simulink model "stellaris_extmode"  (R2014b)
settings: Solver=FixedStepDiscrete  StartTime=0.0  StopTime=10.0  RelTol=1e-3
PreLoadFcn:
  | RTWConfigurationCB('preloadfcn', bdroot);
libraries: stellaris_lib x3, driver_interface_library x2, canblocks_extras x1, targetsExternalModeSwitchLib x1
settings Model: SimulationMode=external  Creator=bas  LastModifiedBy=peselnikmg
settings OptimizationCC: InlineParams=on  OptimizeModelRefInitCode=on  LifeSpan=1
settings DebuggingCC: UnderspecifiedInitializationDetection=Classic  MergeDetectMultiDrivingBlocksExec=none  StateNameClashWarn=warning
settings HardwareCC: ProdEndianess=LittleEndian  ProdHWDeviceType=Texas Instruments->TMS470
settings RTWCC: SystemTargetFile=stellaris.tlc  TemplateMakefile=stellaris_tmf  PostCodeGenCommand=stellaris_customcode(buildInfo)  Description=TI Stellaris LaunchPad  GenerateReport=on  ProcessScript=stellaris_make_rtw_hook  IncludeHyperlinkInReport=on  GenerateTraceInfo=on  GenerateTraceReport=on  GenerateTraceReportSl=on  GenerateTraceReportSf=on  GenerateTraceReportEml=on
settings CodeAppCC: IgnoreCustomStorageClasses=off
settings STFCustomTargetCC: CombineOutputUpdateFcns=on  ERTCustomFileBanners=on  SupportContinuousTime=off  SupportNonInlinedSFcns=off  MATLABClassNameForMDSCustomization=Simulink.SoftwareTarget.ERTCustomization  GRTInterface=off  SystemTargetFile=stellaris.tlc
settings ERTTargetCC: ParMdlRefBuildCompliant=off  CompOptLevelCompliant=off  ConcurrentExecutionCompliant=off  ERTFirstTimeCompliant=off  ModelStepFunctionPrototypeControlCompliant=off  CPPClassGenCompliant=off  GenerateASAP2=on  ExtMode=on  ExtModeTransport=1  ExtModeStaticAllocSize=25000  ExtModeMexFile=stellarisExternalModeOpen  ExtModeMexArgs=1 getpref('stellaris','COMPort') 115200  ExtModeIntrfLevel=Level2  InlinedParameterPlacement=NonHierarchical  ERTCustomFileTemplate=stellaris_main.tlc

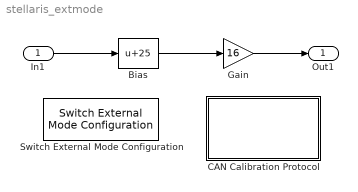
== system stellaris_extmode ==
  In1 : Inport
  Bias : Bias  Bias=25
  CAN Calibration Protocol : Subsystem  InitFcn=|  mask(Stellaris CAN Calibration Protocol){CCP_STATION_ID=hex2dec('1'), module=eCAN_A, ccp_cro_id=hex2dec('6FA'), ccp_cro_message_type=Extended (29-bit identifier), ccp_return_id=hex2dec('6FB'), ccp_return_message_type=Extended (29-bit identifier), TOTAL_NUM_ODTS=8, cro_sample_time=0.1}
      | % START RTW CONFIGURATION CODE %
      | RTWConfigurationCB('rtw_target_initfcn',gcb);
      | % END RTW CONFIGURATION CODE %
      mask prompts: CCP_STATION_ID "CCP station address (16-bit integer):"; module "CAN module:"; ccp_cro_id "CAN message identifier (CRO):"; ccp_cro_message_type "CAN message type (CRO):"; ccp_return_id "CAN message identifier (DTO/DAQ):"; ccp_return_message_type "CAN message type (DTO/DAQ):"; TOTAL_NUM_ODTS "Total Number of Object Descriptor Tables (ODTs):"; cro_sample_time "CRO sample time:"
      mask help:
      | Implements CAN Calibration Protocol (CCP) on the target processor.
      |
      | This block processes Command Receive Object (CRO) messages and outputs the resulting Data Transmission Object (DTO) and Data Acquisition (DAQ) messages.
      mask init:
      | % % Propagate DAQ / DTO message type to underlying blocks
      | % set_param([gcb, '/DAQ Processing/Send DAQ Message/eCAN Transmit'], 'messageType', ccp_return_message_type);
      | % set_param([gcb, '/DTO Processing/CCP(Termination)/CAN Transmit/eCAN Transmit'], 'messageType', ccp_return_message_type);
      | % % Propagate CRO message type to underlying blocks
      | % set_param([gcb, '/eCAN Receive'], 'messageType', ccp_cro_message_type);
      | % % Propagate eCAN module to underlying blocks
      | % set_param([gcb, '/DAQ Processing/Send DAQ Message/eCAN Transmit'], 'useModule', module);
      | % set_param([gcb, '/DTO Processing/CCP(Termination)/CAN Transmit/eCAN Transmit'], 'useModule', module);
      | % set_param([gcb, '/eCAN Receive'], 'useModule', module);
      mask Help: eval('codertarget.internal.helpView(''tic2000'' ,''c280xlibc28xcancalibrationprotocol'')')
      mask TypeOptions module: eCAN_A | eCAN_B
      mask TypeOptions ccp_cro_message_type: Standard (11-bit identifier) | Extended (29-bit identifier)
      mask TypeOptions ccp_return_message_type: Standard (11-bit identifier) | Extended (29-bit identifier)
      mask Display:
      | color('blue');
      | text(0.95, 0.90, 'C28x', ...
      |                 'horizontalalignment', 'right');
      | color('black');
      | text(0.50, 0.12, 'CCP', ...
      |                 'horizontalAlignment','center');
  Gain : Gain  Gain=16
  Switch External Mode Configuration : targetsExternalModeSwitchLib/Switch External Mode Configuration  SystemSampleTime=-1
  Out1 : Outport
  wires:
  In1/1 -> Bias/1
  Bias/1 -> Gain/1
  Gain/1 -> Out1/1

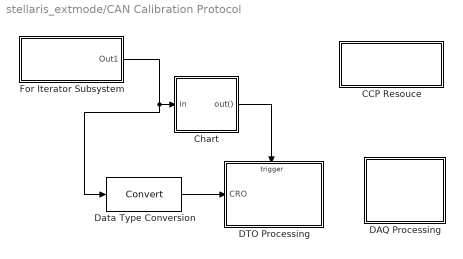
== system stellaris_extmode/CAN Calibration Protocol ==
  CCP Resouce : Subsystem  Tag=RTW CONFIGURATION BLOCK  Priority=-100000  mask{oldParentName=stellaris_extmode/CAN Calibration Protocol, oldBlockName=stellaris_extmode/CAN Calibration Protocol/CCP Resouce, defaultConfigLibrary=}
      mask prompts: oldParentName "Old Parent Name"; oldBlockName "Old Block Name"; defaultConfigLibrary "Default Config Library"
      settings: CopyFcn=RTWConfigurationCB('copyfcn',gcb);  DeleteFcn=RTWConfigurationCB('deletefcn',gcb);  UndoDeleteFcn=RTWConfigurationCB('NameChangeFcn',gcb);  PreSaveFcn=RTWConfigurationCB('presavefcn',gcb);  NameChangeFcn=RTWConfigurationCB('NameChangeFcn',gcb);  OpenFcn=RTWConfigurationCB('openfcn',gcb);
      mask Display: disp('CCP\nResource Block')
  Chart : Stateflow chart  TreatAsAtomicUnit=on
  DAQ Processing : Subsystem
      mask Display: disp('DAQ')
  DTO Processing : Subsystem
      mask Display: disp('DTO')
  Data Type Conversion : DataTypeConversion
  For Iterator Subsystem : Subsystem  TreatAsAtomicUnit=on
  wires:
  Data Type Conversion/1 -> DTO Processing/1(CRO)
  For Iterator Subsystem/1(Out1) -> Chart/1(in), Data Type Conversion/1
  Chart/1(out()) -> DTO Processing/Trigger

== system stellaris_extmode/CAN Calibration Protocol/CCP Resouce ==

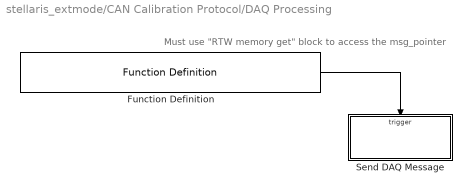
== system stellaris_extmode/CAN Calibration Protocol/DAQ Processing ==
  note: Must use "RTW memory get" block to access the msg_pointer
  Function Definition : driver_interface_library/Function Definition  function_name='void exported_ccp_daq_trigger(uint8_T * msg_pointer)'
  Send DAQ Message : Subsystem  TreatAsAtomicUnit=on
  wires:
  Function Definition/1 -> Send DAQ Message/Trigger

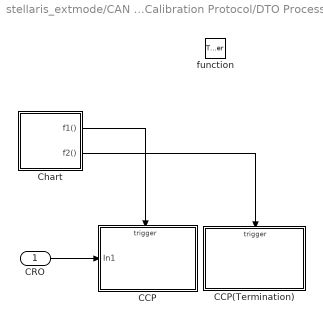
== system stellaris_extmode/CAN Calibration Protocol/DTO Processing ==
  CRO : Inport
  function : TriggerPort  TriggerType=function-call
  CCP : Subsystem
  CCP(Termination) : Subsystem
  Chart : Stateflow chart  TreatAsAtomicUnit=on
  wires:
  Chart/1(f1()) -> CCP/Trigger
  Chart/2(f2()) -> CCP(Termination)/Trigger
  CRO/1 -> CCP/1(In1)

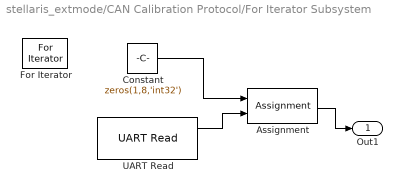
== system stellaris_extmode/CAN Calibration Protocol/For Iterator Subsystem ==
  Assignment : Assignment  OutputInitialize=Specify size for each dimension in table  DiagnosticForDimensions=Warning
  Constant : Constant  Value=zeros(1,8,'int32')
  For Iterator : ForIterator  IterationLimit=8  ShowIterationPort=off
  UART Read : stellaris_lib/UART/UART Read  nbFlag=on
  Out1 : Outport
  wires:
  UART Read/1 -> Assignment/2
  Assignment/1 -> Out1/1
  Constant/1 -> Assignment/1

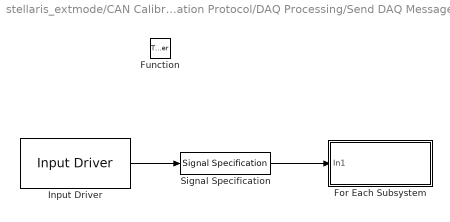
== system stellaris_extmode/CAN Calibration Protocol/DAQ Processing/Send DAQ Message ==
  Function : TriggerPort  TriggerType=function-call
  For Each Subsystem : Subsystem  TreatAsAtomicUnit=on
  Input Driver : driver_interface_library/Input Driver  t=-1  expr='msg_pointer[%<i>]'  portWidth=8  pOpt=[]  expression_type=Not expression
  Signal Specification : SignalSpecification  OutDataTypeStr=uint8
  wires:
  Input Driver/1 -> Signal Specification/1
  Signal Specification/1 -> For Each Subsystem/1(In1)

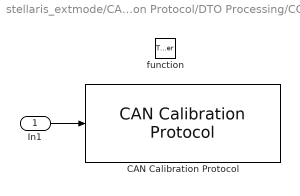
== system stellaris_extmode/CAN Calibration Protocol/DTO Processing/CCP ==
  In1 : Inport
  function : TriggerPort  TriggerType=function-call
  CAN Calibration Protocol : canblocks_extras/CAN Calibration Protocol  CCP_STATION_ID=CCP_STATION_ID  TOTAL_NUM_ODTS=TOTAL_NUM_ODTS  show_commands=off  GET_CCP_VERSIONenabled=on  EXCHANGE_IDenabled=on  SET_MTAenabled=on  DNLOADenabled=on  DNLOAD_6enabled=on  UPLOADenabled=on  SHORT_UPenabled=on  GET_DAQ_SIZEenabled=on  SET_DAQ_PTRenabled=on  WRITE_DAQenabled=on  START_STOPenabled=on  SET_S_STATUSenabled=on  GET_S_STATUSenabled=on  START_STOP_ALLenabled=on
      settings: AttributesFormatString=\n\n
  wires:
  In1/1 -> CAN Calibration Protocol/1

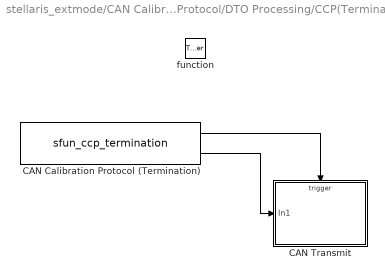
== system stellaris_extmode/CAN Calibration Protocol/DTO Processing/CCP(Termination) ==
  function : TriggerPort  TriggerType=function-call
  CAN Calibration Protocol (Termination) : S-Function  FunctionName=sfun_ccp_termination  EnableBusSupport=off
      mask Display: disp('CCP Termination');
  CAN Transmit : Subsystem
  wires:
  CAN Calibration Protocol (Termination)/2 -> CAN Transmit/1(In1)
  CAN Calibration Protocol (Termination)/1 -> CAN Transmit/Trigger

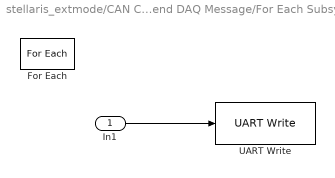
== system stellaris_extmode/CAN Calibration Protocol/DAQ Processing/Send DAQ Message/For Each Subsystem ==
  In1 : Inport  Partition=on  PartitionDimension=1  PartitionWidth=1
  For Each : ForEach  DisableCoverage=on  IndexMode=One-based
  UART Write : stellaris_lib/UART/UART Write  nbFlag=on
  wires:
  In1/1 -> UART Write/1

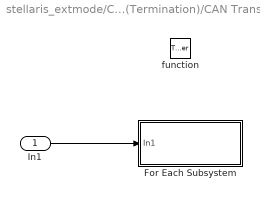
== system stellaris_extmode/CAN Calibration Protocol/DTO Processing/CCP(Termination)/CAN Transmit ==
  In1 : Inport
  function : TriggerPort  TriggerType=function-call
  For Each Subsystem : Subsystem  TreatAsAtomicUnit=on
  wires:
  In1/1 -> For Each Subsystem/1(In1)

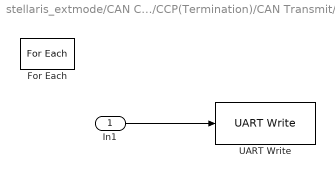
== system stellaris_extmode/CAN Calibration Protocol/DTO Processing/CCP(Termination)/CAN Transmit/For Each Subsystem ==
  In1 : Inport  Partition=on  PartitionDimension=1  PartitionWidth=1
  For Each : ForEach  DisableCoverage=on  IndexMode=One-based
  UART Write : stellaris_lib/UART/UART Write  nbFlag=on
  wires:
  In1/1 -> UART Write/1

== stateflow chart stellaris_extmode/CAN Calibration Protocol/DTO Processing/Chart ==
  (default) -> (junction 2) : {f1,f2}
  events: f1 output FUNCTION_CALL_EVENT; f2 output FUNCTION_CALL_EVENT

== stateflow chart stellaris_extmode/CAN Calibration Protocol/Chart ==
  (default) -> (junction 2) : [in[1]>0]{send(out);}
  data: in input
  events: out output FUNCTION_CALL_EVENT
